simulink model "varios_tanques_r2016a"  (R2016a)
settings: Solver=ode23tb  StartTime=0.0  StopTime=40.0  RelTol=1e-3
settings Model: Creator=Matias  LastModifiedBy=Matias

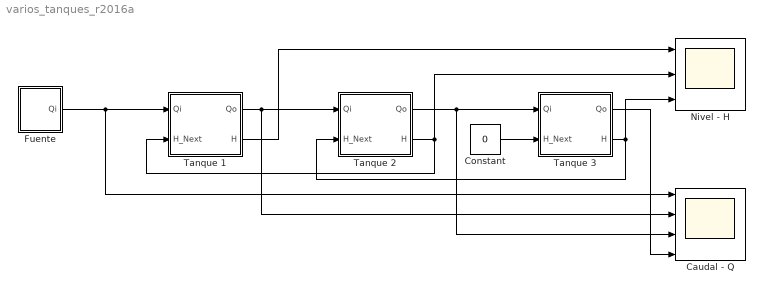
== system varios_tanques_r2016a ==
  Caudal - Q : Scope  NumInputPorts=4
  Constant : Constant  Value=0
  Fuente : Subsystem
  Nivel - H : Scope  NumInputPorts=3
  Tanque 1 : Subsystem
  "Tanque 2 " : Subsystem
  Tanque 3 : Subsystem
  wires:
  Tanque 1/1(Qo) -> Caudal - Q/2, "Tanque 2 "/1("Qi ")
  "Tanque 2 "/2("H ") -> Nivel - H/2, Tanque 1/2(H_Next)
  "Tanque 2 "/1(Qo) -> Caudal - Q/3, Tanque 3/1("Qi ")
  Constant/1 -> Tanque 3/2(H_Next)
  Tanque 3/2("H ") -> Nivel - H/3, "Tanque 2 "/2(H_Next)
  Tanque 1/2("H ") -> Nivel - H/1
  Tanque 3/1(Qo) -> Caudal - Q/4
  Fuente/1(Qi) -> Caudal - Q/1, Tanque 1/1("Qi ")

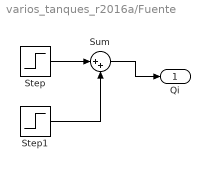
== system varios_tanques_r2016a/Fuente ==
  Step : Step  SampleTime=0
  Step1 : Step  Time=20  After=-1  SampleTime=0
  Sum : Sum  Inputs=|++
  Qi : Outport
  wires:
  Step1/1 -> Sum/2
  Step/1 -> Sum/1
  Sum/1 -> Qi/1

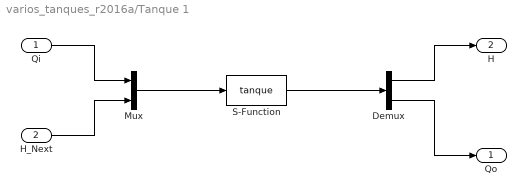
== system varios_tanques_r2016a/Tanque 1 ==
  "Qi " : Inport
  H_Next : Inport  Port=2
  Demux : Demux  Outputs=2
  Mux : Mux  Inputs=2
  S-Function : S-Function  FunctionName=tanque  Parameters=1, 5, 1, 0  SFunctionDeploymentMode=off  EnableBusSupport=off
  Qo : Outport
  "H " : Outport  Port=2
  wires:
  Mux/1 -> S-Function/1
  "Qi "/1 -> Mux/1
  H_Next/1 -> Mux/2
  S-Function/1 -> Demux/1
  Demux/1 -> "H "/1
  Demux/2 -> Qo/1

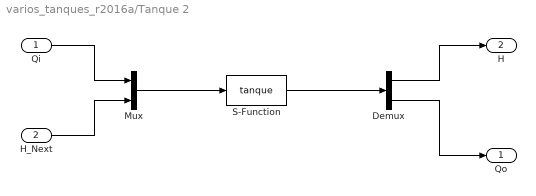
== system varios_tanques_r2016a/Tanque 2  ==
  "Qi " : Inport
  H_Next : Inport  Port=2
  Demux : Demux  Outputs=2
  Mux : Mux  Inputs=2
  S-Function : S-Function  FunctionName=tanque  Parameters=1, 5, 1, 0  SFunctionDeploymentMode=off  EnableBusSupport=off
  Qo : Outport
  "H " : Outport  Port=2
  wires:
  Mux/1 -> S-Function/1
  "Qi "/1 -> Mux/1
  H_Next/1 -> Mux/2
  S-Function/1 -> Demux/1
  Demux/1 -> "H "/1
  Demux/2 -> Qo/1

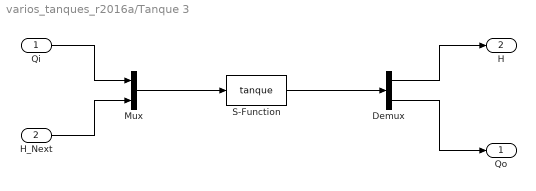
== system varios_tanques_r2016a/Tanque 3 ==
  "Qi " : Inport
  H_Next : Inport  Port=2
  Demux : Demux  Outputs=2
  Mux : Mux  Inputs=2
  S-Function : S-Function  FunctionName=tanque  Parameters=1, 5, 1, 0  SFunctionDeploymentMode=off  EnableBusSupport=off
  Qo : Outport
  "H " : Outport  Port=2
  wires:
  Mux/1 -> S-Function/1
  "Qi "/1 -> Mux/1
  H_Next/1 -> Mux/2
  S-Function/1 -> Demux/1
  Demux/1 -> "H "/1
  Demux/2 -> Qo/1
